simulink library "csc_fdm_feature_detection_matching_lib"  (R2015b)
settings: Solver=ode45  SolverMode=SingleTasking  StartTime=0.0  StopTime=10.0  RelTol=1e-3
values from neighbouring files (symbols this model uses):
  cam_rate_factor_gain = 0    [csc_cam_camera_system_init.m]
undefined symbols (not defined in the file or in its folder): cam_max_rate, KF_DT
libraries: util_common_lib x3, util_info_lib x1, csu_gpe_ground_point_extraction_lib x1
settings Model: Creator=hcannon  LastModifiedBy=jimkaidy
settings DataIOCC: SaveFormat=Array  SignalLoggingSaveFormat=ModelDataLogs
settings OptimizationCC: BlockReduction=off  BooleanDataType=off  ExpressionDepthLimit=2147483647
settings DebuggingCC: SaveWithParameterizedLinksMsg=none  UnderspecifiedInitializationDetection=Classic  MergeDetectMultiDrivingBlocksExec=none  SignalResolutionControl=TryResolveAllWithWarning  FcnCallInpInsideContextMsg=EnableAllAsWarning  StateNameClashWarn=warning  StrictBusMsg=Warning
settings HardwareCC: ProdBitPerPointer=32  ProdLargestAtomicFloat=None  ProdIntDivRoundTo=Undefined  ProdEndianess=Unspecified  ProdWordSize=32  ProdHWDeviceType=32-bit Generic  TargetUnknown=on
settings GRTTargetCC: GeneratePreprocessorConditionals=Disable all  CombineOutputUpdateFcns=off  GRTInterface=on
settings ConfigComp: CovModelRefEnable=Off  CovSFcnEnable=off

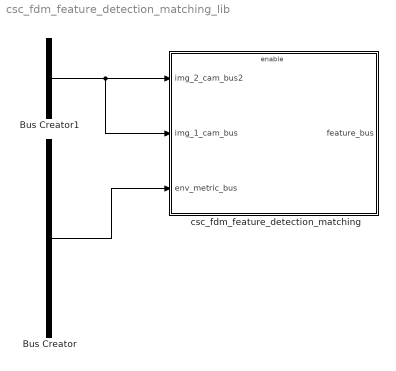
== system csc_fdm_feature_detection_matching_lib ==
  Bus Creator : BusCreator  Inputs=10
  Bus Creator1 : BusCreator  Inputs=5  OutDataTypeStr=Bus: camera_msg  NonVirtualBus=on
  csc_fdm_feature_detection_matching : Subsystem  TreatAsAtomicUnit=on  SystemSampleTime=KF_DT
  wires:
  ? -> Bus Creator/10  "grv_gravity_acc_eci"
  ? -> Bus Creator/1  "rrd_alpha_body_in_eci"
  ? -> Bus Creator/2  "rrk_rate_body_eci_body"
  ? -> Bus Creator/3  "rrk_q_body_from_eci"
  ? -> Bus Creator/4  "rrk_euler_zyx_rot_deg"
  ? -> Bus Creator/5  "rtd_acc_body_in_eci"
  ? -> Bus Creator/6  "rtk_vel_eci"
  ? -> Bus Creator/7  "rtk_pos_eci"
  ? -> Bus Creator/8
  ? -> Bus Creator/9
  Bus Creator1/1 -> csc_fdm_feature_detection_matching/2(img_1_cam_bus), csc_fdm_feature_detection_matching/1(img_2_cam_bus2)
  ? -> Bus Creator1/3  "cam_Cext"
  ? -> Bus Creator1/2  "cam_position_T"
  ? -> Bus Creator1/5  "cam_image_corners"
  ? -> Bus Creator1/4  "cam_projective_P"
  ? -> Bus Creator1/1  "cam_RW2C"
  Bus Creator/1 -> csc_fdm_feature_detection_matching/3(env_metric_bus)

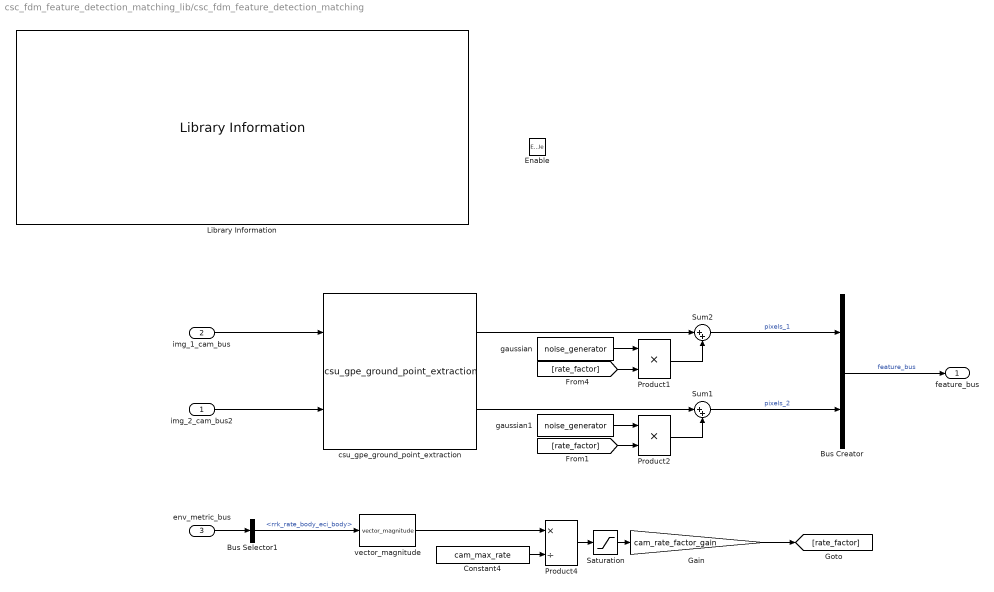
== system csc_fdm_feature_detection_matching_lib/csc_fdm_feature_detection_matching ==
  img_2_cam_bus2 : Inport
  img_1_cam_bus : Inport  Port=2
  env_metric_bus : Inport  Port=3
  Enable : EnablePort
  Bus Creator : BusCreator  Inputs=2
  Bus Selector1 : BusSelector  OutputSignals=lander_state_bus.rrk_rate_body_eci_body
  Constant4 : Constant  Value=cam_max_rate
  Gain : Gain  Gain=cam_rate_factor_gain
  Library Information : util_info_lib/Library Information  owner='NONE'
  Product1 : Product  Inputs=**  RndMeth=Zero
  Product2 : Product  Inputs=**  RndMeth=Zero
  Product4 : Product  Inputs=*/  RndMeth=Zero
  Saturation : Saturate  UpperLimit=10000  LowerLimit=1
  Sum1 : Sum  Inputs=|++
  Sum2 : Sum  Inputs=|++
  csu_gpe_ground_point_extraction : csu_gpe_ground_point_extraction_lib/csu_gpe_ground_point_extraction
  gaussian : util_common_lib/noise_generator  std_dev=cam_pixel_std  bias=cam_pixel_bias  seed=1  on=1  sample_time=sim_time_step_size
  gaussian1 : util_common_lib/noise_generator  std_dev=cam_pixel_std  bias=cam_pixel_bias  seed=1  on=1  sample_time=sim_time_step_size
  vector_magnitude : util_common_lib/vector_magnitude  SystemSampleTime=-1
  feature_bus : Outport
  wires:
  Gain/1 -> [rate_factor]
  Product1/1 -> Sum2/2
  [rate_factor] -> Product1/2
  gaussian/1 -> Product1/1
  Saturation/1 -> Gain/1
  Product4/1 -> Saturation/1
  Constant4/1 -> Product4/2
  vector_magnitude/1 -> Product4/1
  Bus Selector1/1 -> vector_magnitude/1  "<rrk_rate_body_eci_body>"
  Bus Creator/1 -> feature_bus/1  "feature_bus"
  env_metric_bus/1 -> Bus Selector1/1
  img_1_cam_bus/1 -> csu_gpe_ground_point_extraction/1
  img_2_cam_bus2/1 -> csu_gpe_ground_point_extraction/2
  csu_gpe_ground_point_extraction/1 -> Sum2/1
  Product2/1 -> Sum1/2
  [rate_factor] -> Product2/2
  gaussian1/1 -> Product2/1
  csu_gpe_ground_point_extraction/2 -> Sum1/1
  Sum2/1 -> Bus Creator/1  "pixels_1"
  Sum1/1 -> Bus Creator/2  "pixels_2"
